simulink model "LFC_effect_of_Ki"  (R2014a)
settings: Solver=ode45  StartTime=0.0  StopTime=50  RelTol=1e-3
libraries: cstblocks x7
settings Model: Creator=Divya M  LastModifiedBy=Divya M

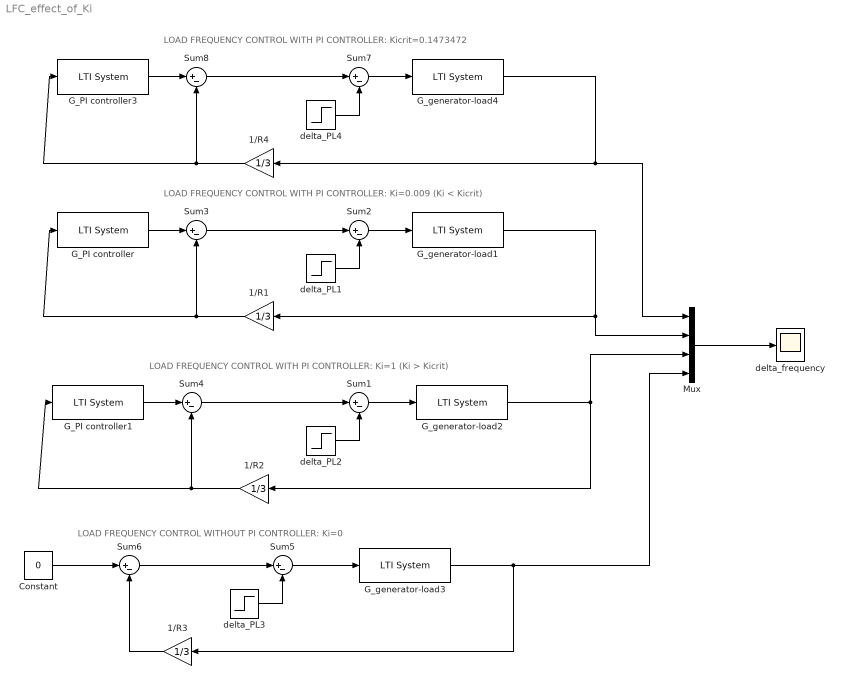
== system LFC_effect_of_Ki ==
  note: LOAD FREQUENCY CONTROL WITH PI CONTROLLER: Ki=0.009 (Ki < Kicrit)
  note: LOAD FREQUENCY CONTROL WITH PI CONTROLLER: Ki=1 (Ki > Kicrit)
  note: LOAD FREQUENCY CONTROL WITHOUT PI CONTROLLER: Ki=0
  note: LOAD FREQUENCY CONTROL WITH PI CONTROLLER: Kicrit=0.1473472
  1/R{1..4} (4 alike) : Gain  Gain=1/3
  Constant : Constant  Value=0
  G_PI controller : cstblocks/LTI System  sys=tf(-0.009,[1 0])  IC=[]
  G_PI controller1 : cstblocks/LTI System  sys=tf(-1,[1 0])  IC=[]
  G_PI controller3 : cstblocks/LTI System  sys=tf(-0.1473472222,[1 0])  IC=[]
  G_generator-load{1..4} (4 alike) : cstblocks/LTI System  sys=tf(100,[20 1])  IC=[]
  Mux : Mux
  Sum{1..8} (8 alike) : Sum  Inputs=|+-
  delta_PL{1..4} (4 alike) : Step  After=0.01  SampleTime=0
  delta_frequency : Scope
      settings: YMin=-0.05  YMax=0.03
  wires:
  Mux/1 -> delta_frequency/1
  Sum2/1 -> G_generator-load1/1
  G_generator-load1/1 -> 1/R1/1, Mux/2
  delta_PL1/1 -> Sum2/2
  1/R1/1 -> G_PI controller/1, Sum3/2
  G_PI controller/1 -> Sum3/1
  Sum1/1 -> G_generator-load2/1
  G_generator-load2/1 -> 1/R2/1, Mux/3
  delta_PL2/1 -> Sum1/2
  1/R2/1 -> G_PI controller1/1, Sum4/2
  G_PI controller1/1 -> Sum4/1
  Sum5/1 -> G_generator-load3/1
  G_generator-load3/1 -> 1/R3/1, Mux/4
  delta_PL3/1 -> Sum5/2
  1/R3/1 -> Sum6/2
  Sum3/1 -> Sum2/1
  Sum4/1 -> Sum1/1
  Sum6/1 -> Sum5/1
  Sum7/1 -> G_generator-load4/1
  G_generator-load4/1 -> Mux/1, 1/R4/1
  delta_PL4/1 -> Sum7/2
  1/R4/1 -> G_PI controller3/1, Sum8/2
  G_PI controller3/1 -> Sum8/1
  Sum8/1 -> Sum7/1
  Constant/1 -> Sum6/1
